simulink model "Copy_of_lqg"  (R2022a)
settings: Solver=VariableStepAuto  StartTime=0.0  StopTime=10  RelTol=1e-3
values from neighbouring files (symbols this model uses):
  Ad = sysd.a    [LQG_2by2_sim.m]
  Bd = sysd.b    [LQG_2by2_sim.m]
  K = (4-3*rho+q)./(8+10*rho+2*q)    [kalman_example.m]
undefined symbols (not defined in the file or in its folder): Cd, Kr, L, Ts, var_Te, var_v1, var_v2, var_va
libraries: SignalEditorBlockLib x1
settings Model: Creator=lplal  LastModifiedBy=Ccm

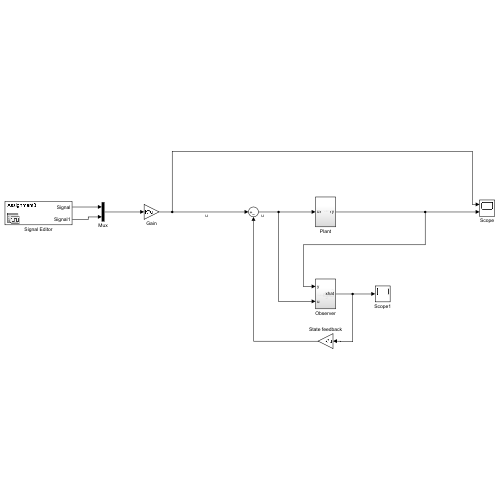
[thumbnail: Simulink's stored preview of the top-level diagram]
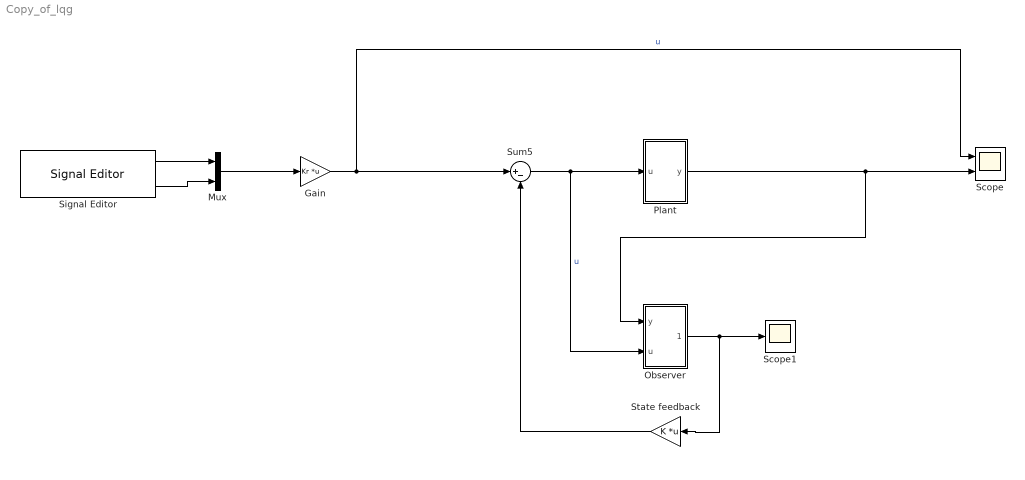
== system Copy_of_lqg ==
  Gain : Gain  Gain=Kr  Multiplication=Matrix(K*u)
  Mux : Mux  Inputs=2
  Observer : Subsystem
  Plant : Subsystem
  Scope : Scope  NumInputPorts=2
  Scope1 : Scope
  Signal Editor : SignalEditorBlockLib/Signal Editor  FileName=signal.mat  ActiveScenario=Assignment3  ActiveSignal=Signal  IsBus=off  OutputBusObjectStr=Bus: <object name>  SampleTime=0  Interpolate=off  ZeroCross=off  OutputAfterFinalValue=Setting to zero  Unit=inherit  PreserveSignalName=on
  State feedback : Gain  Gain=K  Multiplication=Matrix(K*u)
  Sum5 : Sum  Inputs=|+-
  wires:
  Sum5/1 -> Observer/2(u), Plant/1(u)  "u"
  State feedback/1 -> Sum5/2
  Observer/1(xhat) -> Scope1/1, State feedback/1
  Plant/1(y) -> Scope/2, Observer/1(y)
  Gain/1 -> Sum5/1, Scope/1  "u"
  Signal Editor/1 -> Mux/1
  Signal Editor/2 -> Mux/2
  Mux/1 -> Gain/1

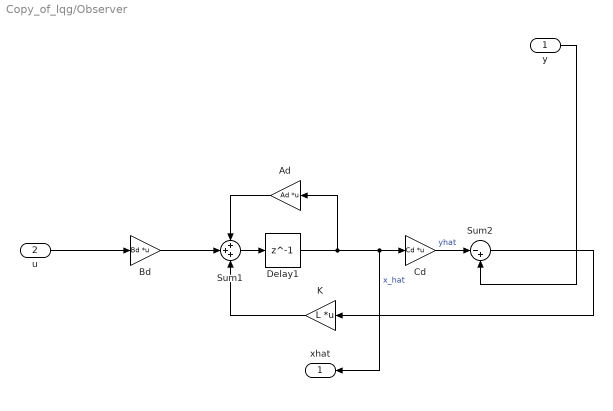
== system Copy_of_lqg/Observer ==
  y : Inport
  u : Inport  Port=2
  Ad : Gain  Gain=Ad  Multiplication=Matrix(K*u)
  Bd : Gain  Gain=Bd  Multiplication=Matrix(K*u)
  Cd : Gain  Gain=Cd  Multiplication=Matrix(K*u)
  Delay1 : Delay  DelayLength=1
  K : Gain  Gain=L  Multiplication=Matrix(K*u)
  Sum1 : Sum  Inputs=+++
  Sum2 : Sum  Inputs=|-+
  xhat : Outport
  wires:
  Ad/1 -> Sum1/1
  Sum1/1 -> Delay1/1
  Sum2/1 -> K/1
  u/1 -> Bd/1
  Bd/1 -> Sum1/2
  y/1 -> Sum2/2
  K/1 -> Sum1/3
  Delay1/1 -> Ad/1, xhat/1, Cd/1  "x_hat"
  Cd/1 -> Sum2/1  "yhat"

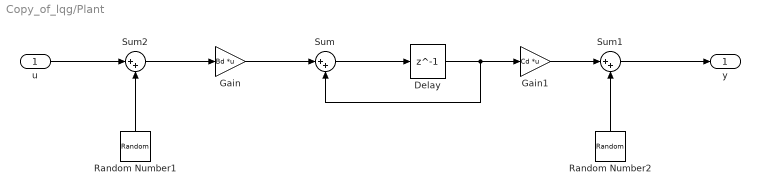
== system Copy_of_lqg/Plant ==
  u : Inport
  Delay : Delay  DelayLength=1  InitialCondition=0
  Gain : Gain  Gain=Bd  Multiplication=Matrix(K*u)
  Gain1 : Gain  Gain=Cd  Multiplication=Matrix(K*u)
  Random Number1 : RandomNumber  Variance=[var_va,var_Te]  SampleTime=Ts
  Random Number2 : RandomNumber  Variance=[var_v1,var_v2]  SampleTime=Ts
  Sum : Sum  Inputs=|++
  Sum1 : Sum  Inputs=|++
  Sum2 : Sum  Inputs=|++
  y : Outport
  wires:
  Sum2/1 -> Gain/1
  Sum1/1 -> y/1
  Sum/1 -> Delay/1
  Delay/1 -> Sum/2, Gain1/1
  Random Number2/1 -> Sum1/2
  Random Number1/1 -> Sum2/2
  u/1 -> Sum2/1
  Gain/1 -> Sum/1
  Gain1/1 -> Sum1/1
